simulink model "final_project"  (R2021a)
settings: Solver=VariableStepAuto  StartTime=0.0  StopTime=inf  RelTol=1e-3
libraries: vrlib x1
settings Model: Creator=kbhar  LastModifiedBy=kbhar

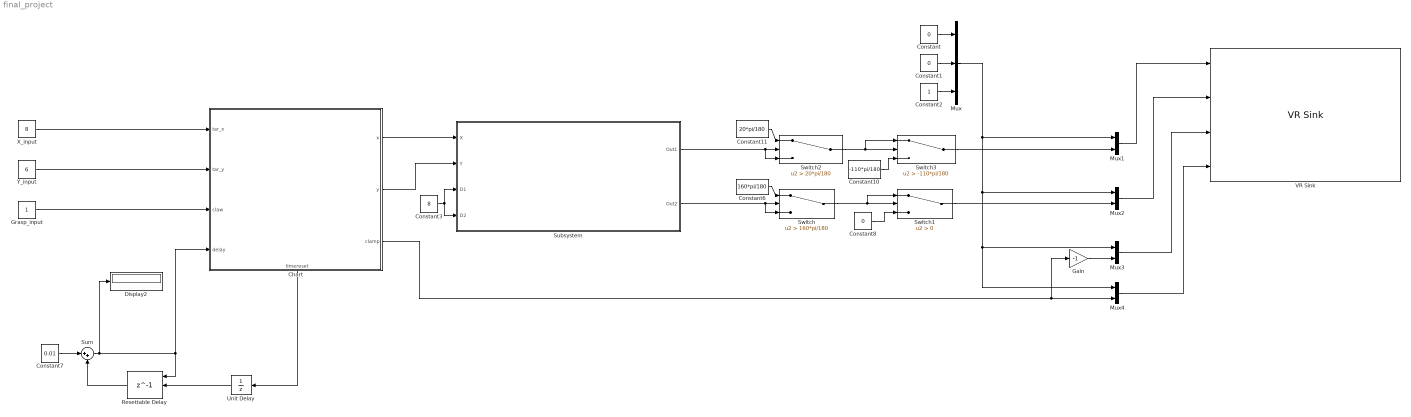
== system final_project ==
  Chart : Stateflow chart  TreatAsAtomicUnit=on
      settings: PortSchema="{\"entries\":[{\"content\":{\"sides\":[{\"content\":{\"connectorIds\":[\"In1\",\"In2\",\"In4\",\"In3\"]},\"type\":\"ConnectorPlacement.EquallySpacedRectSide\",\"uuid\":\"972cd691-1960-4212-a7ac-9137271643fd\"},{\"content\":{\"connectorIds\":[\"Out1\",\"Out2\",\"Out3\"],\"side\":\"RIGHT\"},\"type\":\"ConnectorPlacement.EquallySpacedRectSide\",\"uuid\":\"f459904b-1352-4c88-9dc5-145db930a385\"},{\"content\":{\"connectorIds\":[],\"side\":\"TOP\"},\"type\":\"ConnectorPlacement.EquallySpacedRectSide\",\"uuid\":\"43801eda-f3fa-4c23-9103-228be10a1c76\"},{\"content\":{\"connectorIds\":[\"Out4\"],\"side\":\"BOTTOM\"},\"type\":\"ConnectorPlacement.EquallySpacedRectSide\",\"uuid\":\"6b83d1f9-b36a-42f2-8968-91e63af5868d\"}]},\"type\":\"ConnectorPlacement.EquallySpacedConnector\",\"uuid\":\"8f8af6c6-e99e-43c9-b621-3410c3268dba\"}],\"packageUris\":[\"http://schema.mathworks.com/mf0/Connector/R2020b\"],\"version\":\"1.0\"}"
  Constant : Constant  Value=0
  Constant1 : Constant  Value=0
  Constant10 : Constant  Value=-110*pi/180
  Constant11 : Constant  Value=20*pi/180
  Constant2 : Constant
  Constant3 : Constant  Value=8
  Constant6 : Constant  Value=160*pi/180
  Constant7 : Constant  Value=0.01
  Constant8 : Constant  Value=0
  Display2 : Display
  Gain : Gain  Gain=-1
  Grasp_input : Constant
  Mux : Mux  Inputs=3
  Mux{1..4} (4 alike) : Mux  Inputs=2
  Resettable Delay : Delay  DelayLength=1  InitialConditionSource=Input port  ExternalReset=Rising
      settings: InputPortMap=u0,r5,p4
  Subsystem : Subsystem
  Sum : Sum  Inputs=|++
  Switch : Switch  Criteria=u2 > Threshold  Threshold=160*pi/180
  Switch1 : Switch  Criteria=u2 > Threshold
  Switch2 : Switch  Criteria=u2 > Threshold  Threshold=20*pi/180
  Switch3 : Switch  Criteria=u2 > Threshold  Threshold=-110*pi/180
  Unit Delay : UnitDelay  SampleTime=-1  HasFrameUpgradeWarning=on
  VR Sink : vrlib/VR Sink  InstantiateOnLoad=on  SampleTime=0.1  ViewEnable=on  RemoteChange=off  RemoteView=off  FieldsWritten=j1.rotation.4.1.1.double#j2.rotation.4.1.1.double#claw1_j.rotation.4.1.1.double#claw2_j.rotation.4.1.1.double  WorldFileName=C:\Bharat\College\Projects\Arm Control\Files\final_project.wrl  AutoView=off  VideoDimensions=[]  AllowVariableSize=off  FigureProperties="{'Position', 'Name', 'Viewpoint', 'CameraBound', 'CameraDirection', 'CameraPosition', 'CameraUpVector', 'ZoomFactor', 'Antialiasing', 'Headlight', 'Lighting', 'NavPanel', 'Sound', 'StatusBar', 'Stereo3D', 'Stereo3DCameraOffset', 'Stereo3DHIT', 'ToolBar', 'Textures', 'Transparency', 'Triad', 'Wireframe', 'NavZones', 'NavMode', 'NavSpeed', 'CaptureFileFormat', 'CaptureFileName', 'Record2DCompressMethod', 'Record2DCompressQuality', 'Record2D', 'Record2DFileName', 'Record2DFPS'; [3.9060000000000002e+02   2.5020000000000005e+02   5.7600000000000000e+02   3.5000000000000000e+02], '', '', 'on', [1.7285373096757889e-01   0.0000000000000000e+00  -9.8494750504307993e-01], [-7.7018901396345454e+00   2.0137848854064941e+00   5.3886570655346766e+01], [0.0000000000000000e+00   1.0000000000000000e+00   0.0000000000000000e+00], [1.0000000000000000e+00], 'on', 'on', 'on', 'halfbar', 'on', 'on', 'off', [1.0000000149011612e-01], [0.0000000000000000e+00], 'on', 'on', 'on', 'none', 'off', 'off', 'fly', 'normal', 'tif', '%f_anim_%n.tif', 'auto', [7.5000000000000000e+01], 'off', '%f_anim_%n.avi', 'auto'}"
  X_input : Constant  Value=8
  Y_input : Constant  Value=6
  wires:
  Constant/1 -> Mux/1
  Constant1/1 -> Mux/2
  Constant2/1 -> Mux/3
  Constant3/1 -> Subsystem/4(D2), Subsystem/3(D1)
  Mux/1 -> Mux4/1, Mux3/1, Mux2/1, Mux1/1
  Subsystem/2(Out2) -> Switch/3, Switch/2
  Chart/1(x) -> Subsystem/1(X)
  Chart/2(y) -> Subsystem/2(Y)
  X_input/1 -> Chart/1(tar_x)
  Y_input/1 -> Chart/2(tar_y)
  Chart/3(clamp) -> Mux4/2, Gain/1
  Gain/1 -> Mux3/2
  Chart/4(timereset) -> Unit Delay/1
  Sum/1 -> Resettable Delay/1, Chart/3(delay), Display2/1
  Constant7/1 -> Sum/1
  Resettable Delay/1 -> Sum/2
  Unit Delay/1 -> Resettable Delay/2
  Switch/1 -> Switch1/2, Switch1/1
  Constant6/1 -> Switch/1
  Constant8/1 -> Switch1/3
  Switch1/1 -> Mux2/2
  Constant10/1 -> Switch3/3
  Constant11/1 -> Switch2/1
  Switch2/1 -> Switch3/2, Switch3/1
  Subsystem/1(Out1) -> Switch2/2, Switch2/3
  Switch3/1 -> Mux1/2
  Mux1/1 -> VR Sink/1
  Mux2/1 -> VR Sink/2
  Mux3/1 -> VR Sink/3
  Mux4/1 -> VR Sink/4
  Grasp_input/1 -> Chart/4(claw)

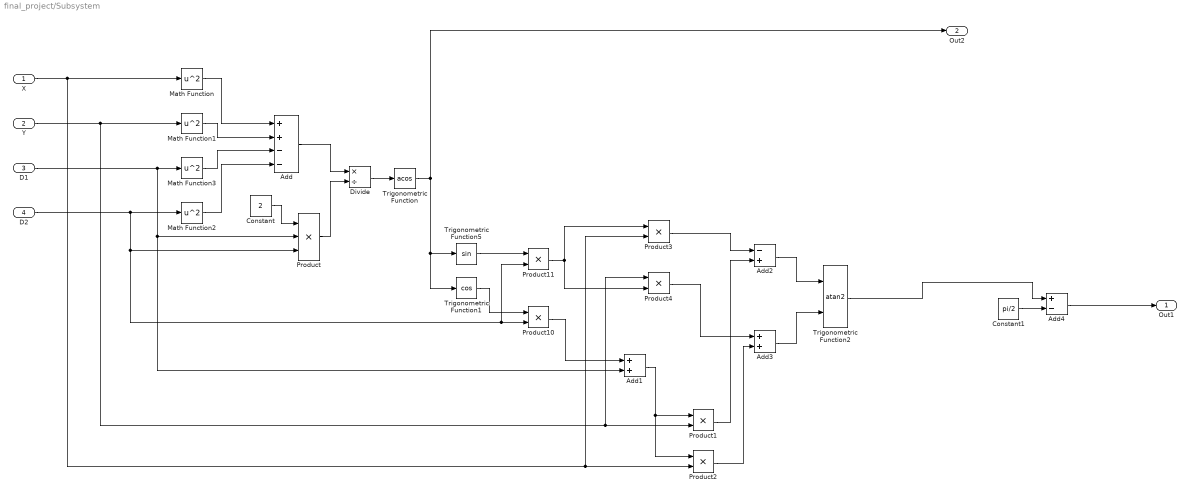
== system final_project/Subsystem ==
  X : Inport
  Y : Inport  Port=2
  D1 : Inport  Port=3
  D2 : Inport  Port=4
  Add : Sum  Inputs=++--
  Add1 : Sum
  Add2 : Sum  Inputs=-+
  Add3 : Sum
  Add4 : Sum  Inputs=+-
  Constant : Constant  Value=2
  Constant1 : Constant  Value=pi/2
  Divide : Product  Inputs=*/
  Math Function{,1..3} (4 alike) : Math  Operator=square  SaturateOnIntegerOverflow=on
  Product : Product  Inputs=3
  Product{1..4,10..11} (6 alike) : Product
  Trigonometric Function : Trigonometry  Operator=acos
  Trigonometric Function1 : Trigonometry  Operator=cos
  Trigonometric Function2 : Trigonometry  Operator=atan2
  Trigonometric Function5 : Trigonometry
  Out1 : Outport
  Out2 : Outport  Port=2
  wires:
  Trigonometric Function1/1 -> Product10/1
  D1/1 -> Add1/2, Product/2, Math Function3/1
  Math Function2/1 -> Add/4
  Trigonometric Function5/1 -> Product11/1
  X/1 -> Product2/2, Product3/2, Math Function/1
  Product/1 -> Divide/2
  Math Function3/1 -> Add/3
  Add/1 -> Divide/1
  Math Function1/1 -> Add/2
  Product2/1 -> Add3/2
  Product11/1 -> Product3/1, Product4/2
  Product1/1 -> Add2/2
  Add2/1 -> Trigonometric Function2/1
  Divide/1 -> Trigonometric Function/1
  Product3/1 -> Add2/1
  D2/1 -> Math Function2/1, Product11/2, Product10/2, Product/3
  Add1/1 -> Product1/1, Product2/1
  Math Function/1 -> Add/1
  Product10/1 -> Add1/1
  Product4/1 -> Add3/1
  Constant/1 -> Product/1
  Add3/1 -> Trigonometric Function2/2
  Y/1 -> Product1/2, Product4/1, Math Function1/1
  Add4/1 -> Out1/1
  Constant1/1 -> Add4/2
  Trigonometric Function2/1 -> Add4/1
  Trigonometric Function/1 -> Out2/1, Trigonometric Function1/1, Trigonometric Function5/1

== stateflow chart final_project/Chart ==
  state start_state
    clamp = 0; x = 0; y = 0;
    timereset = 0;
  state centre_position
    clamp = 0; x = 0; y = 0;
    timereset = 1;
  state hold
    clamp = 0; x = 0; y = 0;
    timereset = 0;
  state target_position
    x = x + 0.0005*tar_x; y = y + 0.0005*tar_y;
  state hold1
    x = tar_x; y = tar_y;
  state grasp
    clamp = clamp + 0.01;
  state hold2
    clamp = 1.571;
  (default) -> start_state
  start_state -> centre_position
  hold2 -> centre_position : [delay>50]
  hold1 -> centre_position [order 2] : [claw ~= 1 & delay > 45]
  centre_position -> hold
  hold -> target_position : [delay>10]
  target_position -> target_position [order 2] : [x<tar_x]
  target_position -> hold1 [order 1] : [x >= tar_x & y>=tar_y]
  hold1 -> grasp [order 1] : [claw == 1]
  grasp -> grasp [order 2] : [clamp < 1.571]
  grasp -> hold2 [order 1] : [clamp >= 1.571]
  data: x output; y output; tar_x input; tar_y input; clamp output; delay input; timereset output; claw input
